simulink model "cw1_sim"  (R2023b)
settings: Solver=ode45  StartTime=0.0  StopTime=300e-3  MaxStep=1e-3  RelTol=1e-3
settings Model: Creator=rolni  LastModifiedBy=rolni

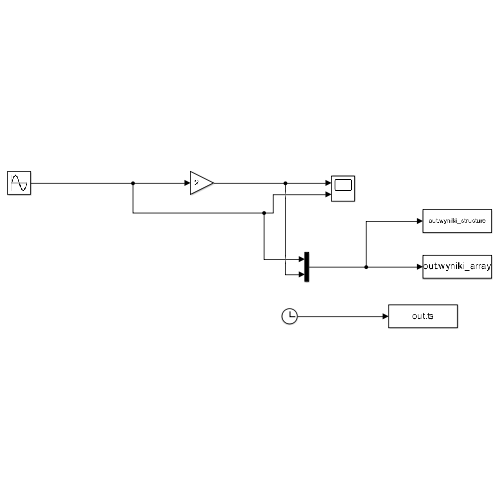
[thumbnail: Simulink's stored preview of the top-level diagram]
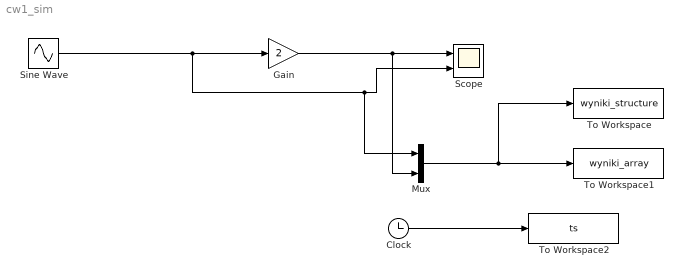
== system cw1_sim ==
  Clock : Clock
  Gain : Gain  Gain=2
  Mux : Mux  Inputs=2
  Scope : Scope  NumInputPorts=2
  Sine Wave : Sin  Frequency=314.159265  SampleTime=0
  To Workspace : ToWorkspace  VariableName=wyniki_structure  SaveFormat=Structure With Time  SampleTime=-1
  To Workspace1 : ToWorkspace  VariableName=wyniki_array  SampleTime=-1
  To Workspace2 : ToWorkspace  VariableName=ts  SaveFormat=Timeseries  SampleTime=-1
  wires:
  Sine Wave/1 -> Mux/1, Scope/2, Gain/1
  Gain/1 -> Mux/2, Scope/1
  Mux/1 -> To Workspace1/1, To Workspace/1
  Clock/1 -> To Workspace2/1
